simulink model "Model_DiscreteSSRedOrderNominalTrackingSystem"  (R2024b)
settings: Solver=ode45  StartTime=0.0  StopTime=5  RelTol=1e-3
values from neighbouring files (symbols this model uses):
  Ts = Ts_values(i)    [A_final_measurements.m]    (also in Plant_EstimTrialUpdateLAB17_04_25.m = 0.001)
settings Model: Creator=Riccardo Grosso  LastModifiedBy=Buton

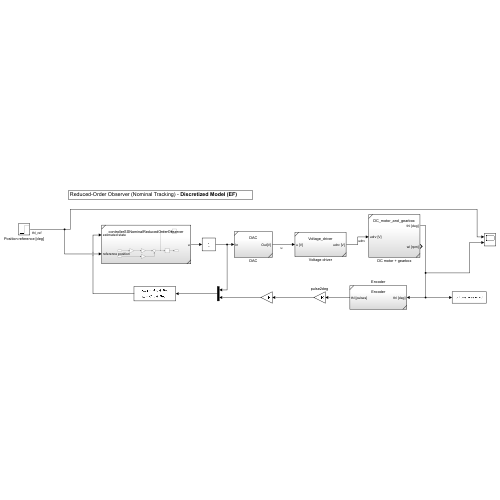
[thumbnail: Simulink's stored preview of the top-level diagram]
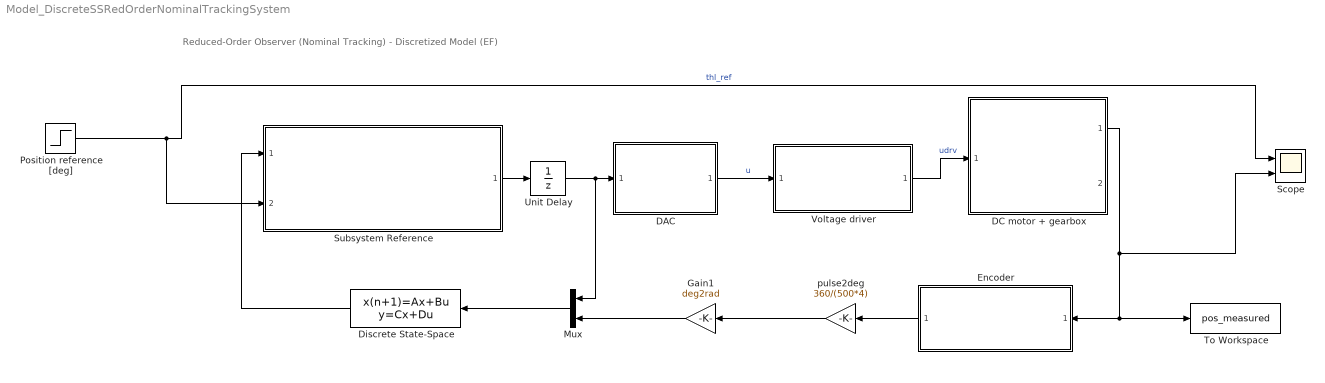
== system Model_DiscreteSSRedOrderNominalTrackingSystem ==
  note: Reduced-Order Observer (Nominal Tracking) - Discretized Model (EF)
  DAC : Subsystem  ReferencedSubsystem=DAC
  DC motor + gearbox : Subsystem  ReferencedSubsystem=DC_motor_and_gearbox
  Discrete State-Space : DiscreteStateSpace  A=-0.617518353278843  B=[4.60319351098823 -1076.45747529499]  C=[0;0.0427627481107283]  D=[0 1;0.514652680207781 28.4585827262108]  SampleTime=Ts
  Encoder : Subsystem  ReferencedSubsystem=Encoder
  Gain1 : Gain  Gain=deg2rad
  Mux : Mux  Inputs=2
  Position reference [deg] : Step  Time=0  After=50  SampleTime=0
  Scope : Scope  NumInputPorts=2
  Subsystem Reference : Subsystem  ReferencedSubsystem=controllerSSNominalReducedOrderObserver
  To Workspace : ToWorkspace  VariableName=pos_measured  SaveFormat=Timeseries  SampleTime=-1
  Unit Delay : UnitDelay  SampleTime=-1  HasFrameUpgradeWarning=on
  Voltage driver : Subsystem  ReferencedSubsystem=Voltage_driver
  pulse2deg : Gain  Gain=360/(500*4)
  wires:
  DAC/1 -> Voltage driver/1  "u"
  Voltage driver/1 -> DC motor + gearbox/1  "udrv"
  Encoder/1 -> pulse2deg/1
  DC motor + gearbox/1 -> Scope/2, Encoder/1, To Workspace/1
  Position reference [deg]/1 -> Subsystem Reference/2, Scope/1  "thl_ref"
  Subsystem Reference/1 -> Unit Delay/1
  pulse2deg/1 -> Gain1/1
  Gain1/1 -> Mux/2
  Discrete State-Space/1 -> Subsystem Reference/1
  Mux/1 -> Discrete State-Space/1
  Unit Delay/1 -> Mux/1, DAC/1
